simulink model "wlan_phy_tx_pmd"  (Simulink 7.8)
settings: Solver=ode45  StartTime=0.0  StopTime=17e3  RelTol=1e-3
PostLoadFcn:
  | wlan_phy_tx_init
InitFcn:
  | wlan_phy_tx_init
StartFcn:
  | wlan_phy_tx_init
undefined symbols (not defined in the file): gcbh, interleave_16QAM, interleave_64QAM_addr, interleave_bpsk, interleave_QPSK, MAX_NUM_BYTES, MAX_NUM_SC, Mod_Constellation_16QAM, Mod_Constellation_64QAM, Mod_Constellation_BPSK, Mod_Constellation_QPSK, Preamble_IQ, xlBlockLoadCallback, xlGetNormalizedPeriod
libraries: xbsIndex_r4 x1164, xbsEDKLib_r4 x1
(part 4 of 8)

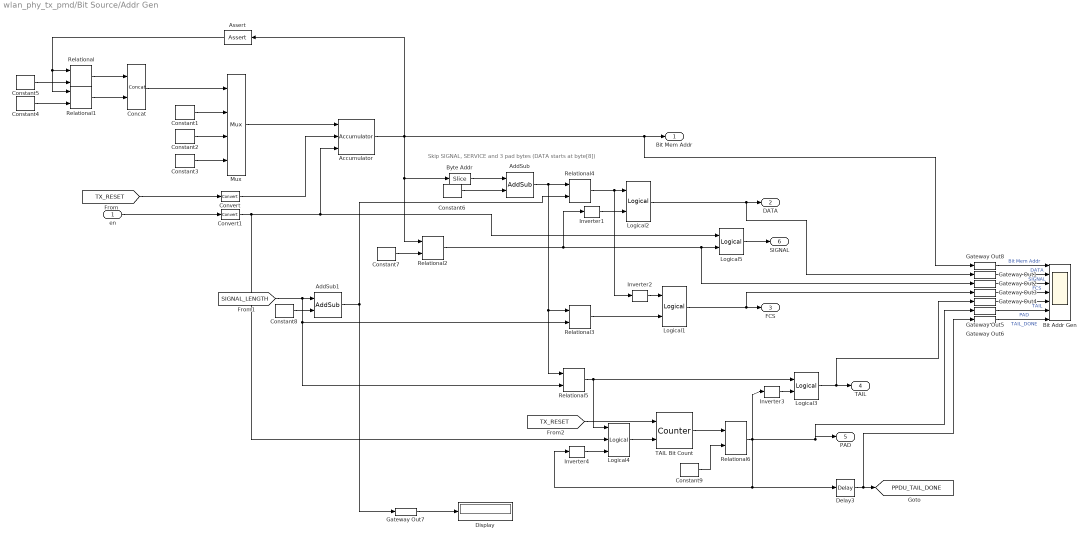
== system wlan_phy_tx_pmd/Bit Source/Addr Gen ==
  note: Skip SIGNAL, SERVICE and
      | 3 pad bytes
      | (DATA starts at byte[8])
  en : Inport
  Accumulator : xbsIndex_r4/Accumulator  operation=Add  n_bits=3 + ceil(log2(MAX_NUM_BYTES))  overflow=Wrap  scale=1  rst=on  infoeditControl=reset for floating point data type must be asserted for a minimum of 2 cycles  hasbypass=off  en=on  latency=0  dbl_ovrd=off  msb_inp=100  msb=100  lsb=-100  use_behavioral_HDL=on  implementation=Fabric  block_type=accum
  AddSub : xbsIndex_r4/AddSub  mode=Subtraction  use_carryin=off  use_carryout=off  en=off  latency=0  precision=User Defined  arith_type=Unsigned  n_bits=ceil(log2(MAX_NUM_BYTES))  bin_pt=0  quantization=Truncate  overflow=Saturate  dbl_ovrd=off  use_behavioral_HDL=off  hw_selection=Fabric  pipelined=off  block_type=addsub
  AddSub1 : xbsIndex_r4/AddSub  mode=Subtraction  use_carryin=off  use_carryout=off  en=off  latency=0  precision=User Defined  arith_type=Unsigned  n_bits=ceil(log2(MAX_NUM_BYTES))  bin_pt=0  quantization=Truncate  overflow=Saturate  dbl_ovrd=off  use_behavioral_HDL=off  hw_selection=Fabric  pipelined=off  block_type=addsub
  Assert : xbsIndex_r4/Assert  assert_type=off  type_source=Explicitly  gui_display_data_type=Fixed-point  arith_type="Signed  (2's comp)"  n_bits=16  bin_pt=14  preci_type=Single  exp_width=8  frac_width=24  assert_rate=on  rate_source=Explicitly  period=1  output_port=on  block_type=assert
  Bit Addr Gen : Scope  NumInputPorts=7
      settings: TimeRange=10000  YMin=0~0~0~0~0~0~0  YMax=1~1~1~1~25~1~1  SaveName=ScopeData8
  Byte Addr : xbsIndex_r4/Slice  nbits=ceil(log2(MAX_NUM_BYTES))  boolean_output=off  mode=Upper Bit Location + Width  bit1=0  base1=MSB of Input  bit0=0  base0=LSB of Input  dbl_ovrd=off  block_type=slice
  Concat : xbsIndex_r4/Concat  num_inputs=2  dbl_ovrd=off  block_type=concat
  Constant1 : xbsIndex_r4/Constant  const=1  gui_display_data_type=Fixed-point  arith_type=Unsigned  n_bits=2  bin_pt=0  preci_type=Single  exp_width=8  frac_width=24  explicit_period=off  period=1  equ=P=C  opselect=C  inp2=PCIN>>17  opr=+  inp1=P  carry=CIN  dbl_ovrd=off  block_type=constant
  Constant2 : xbsIndex_r4/Constant  const=9  gui_display_data_type=Fixed-point  arith_type=Unsigned  n_bits=4  bin_pt=0  preci_type=Single  exp_width=8  frac_width=24  explicit_period=off  period=1  equ=P=C  opselect=C  inp2=PCIN>>17  opr=+  inp1=P  carry=CIN  dbl_ovrd=off  block_type=constant
  Constant3 : xbsIndex_r4/Constant  const=17  gui_display_data_type=Fixed-point  arith_type=Unsigned  n_bits=5  bin_pt=0  preci_type=Single  exp_width=8  frac_width=24  explicit_period=off  period=1  equ=P=C  opselect=C  inp2=PCIN>>17  opr=+  inp1=P  carry=CIN  dbl_ovrd=off  block_type=constant
  Constant4 : xbsIndex_r4/Constant  const=23  gui_display_data_type=Fixed-point  arith_type=Unsigned  n_bits=5  bin_pt=0  preci_type=Single  exp_width=8  frac_width=24  explicit_period=off  period=1  equ=P=C  opselect=C  inp2=PCIN>>17  opr=+  inp1=P  carry=CIN  dbl_ovrd=off  block_type=constant
  Constant5 : xbsIndex_r4/Constant  const=47  gui_display_data_type=Fixed-point  arith_type=Unsigned  n_bits=6  bin_pt=0  preci_type=Single  exp_width=8  frac_width=24  explicit_period=off  period=1  equ=P=C  opselect=C  inp2=PCIN>>17  opr=+  inp1=P  carry=CIN  dbl_ovrd=off  block_type=constant
  Constant6 : xbsIndex_r4/Constant  const=8  gui_display_data_type=Fixed-point  arith_type=Unsigned  n_bits=4  bin_pt=0  preci_type=Single  exp_width=8  frac_width=24  explicit_period=off  period=1  equ=P=C  opselect=C  inp2=PCIN>>17  opr=+  inp1=P  carry=CIN  dbl_ovrd=off  block_type=constant
  Constant7 : xbsIndex_r4/Constant  const=24  gui_display_data_type=Fixed-point  arith_type=Unsigned  n_bits=5  bin_pt=0  preci_type=Single  exp_width=8  frac_width=24  explicit_period=off  period=1  equ=P=C  opselect=C  inp2=PCIN>>17  opr=+  inp1=P  carry=CIN  dbl_ovrd=off  block_type=constant
  Constant8 : xbsIndex_r4/Constant  const=4  gui_display_data_type=Fixed-point  arith_type=Unsigned  n_bits=3  bin_pt=0  preci_type=Single  exp_width=8  frac_width=24  explicit_period=off  period=1  equ=P=C  opselect=C  inp2=PCIN>>17  opr=+  inp1=P  carry=CIN  dbl_ovrd=off  block_type=constant
  Constant9 : xbsIndex_r4/Constant  const=5  gui_display_data_type=Fixed-point  arith_type=Unsigned  n_bits=3  bin_pt=0  preci_type=Single  exp_width=8  frac_width=24  explicit_period=off  period=1  equ=P=C  opselect=C  inp2=PCIN>>17  opr=+  inp1=P  carry=CIN  dbl_ovrd=off  block_type=constant
  Convert : xbsIndex_r4/Convert  gui_display_data_type=Boolean  arith_type=Boolean  n_bits=16  bin_pt=14  float_type=Single  exp_bits=8  fraction_bits=24  quantization=Truncate  overflow=Wrap  en=off  latency=0  dbl_ovrd=off  pipeline=off  block_type=convert
  Convert1 : xbsIndex_r4/Convert  gui_display_data_type=Boolean  arith_type=Boolean  n_bits=16  bin_pt=14  float_type=Single  exp_bits=8  fraction_bits=24  quantization=Truncate  overflow=Wrap  en=off  latency=0  dbl_ovrd=off  pipeline=off  block_type=convert
  Delay3 : xbsIndex_r4/Delay  rst=off  infoeditControl=Selection of Reset will increase slice count due to use of real FFs and instead of SRLs  en=off  latency=1  dbl_ovrd=off  reg_retiming=off  block_type=delay
  Display : Display
  Gateway Out{1..8} (8 alike) : xbsIndex_r4/Gateway Out  inherit_from_input=off  hdl_port=off  timing_constraint=None  locs_specified=off  LOCs={}  UseAsDAC=off  DACChannel='1'  block_type=gatewayout
  Inverter{1..4} (4 alike) : xbsIndex_r4/Inverter  en=off  latency=0  dbl_ovrd=off  block_type=inv
      settings: xl_area=[0 0 0 0 0 0 0]  block_version=VER_STRING_GOES_HERE
  Logical{1..3,5} (4 alike) : xbsIndex_r4/Logical  logical_function=AND  inputs=2  en=off  latency=0  precision=Full  arith_type=Unsigned  n_bits=16  bin_pt=0  align_bp=on  dbl_ovrd=off  block_type=logical
  Logical4 : xbsIndex_r4/Logical  logical_function=AND  inputs=3  en=off  latency=0  precision=Full  arith_type=Unsigned  n_bits=16  bin_pt=0  align_bp=on  dbl_ovrd=off  block_type=logical
  Mux : xbsIndex_r4/Mux  inputs=3  en=off  latency=0  precision=Full  arith_type=Unsigned  n_bits=16  bin_pt=14  quantization=Truncate  overflow=Wrap  dbl_ovrd=off  block_type=mux
  Relational : xbsIndex_r4/Relational  mode=a=b  en=off  latency=0  dbl_ovrd=off  block_type=relational
  Relational1 : xbsIndex_r4/Relational  mode=a=b  en=off  latency=0  dbl_ovrd=off  block_type=relational
  Relational2 : xbsIndex_r4/Relational  mode=a<b  en=off  latency=0  dbl_ovrd=off  block_type=relational
  Relational3 : xbsIndex_r4/Relational  mode=a<b  en=off  latency=0  dbl_ovrd=off  block_type=relational
  Relational4 : xbsIndex_r4/Relational  mode=a<b  en=off  latency=0  dbl_ovrd=off  block_type=relational
  Relational5 : xbsIndex_r4/Relational  mode=a>=b  en=off  latency=0  dbl_ovrd=off  block_type=relational
  Relational6 : xbsIndex_r4/Relational  mode=a>b  en=off  latency=0  dbl_ovrd=off  block_type=relational
  TAIL Bit Count : xbsIndex_r4/Counter  cnt_type=Count Limited  cnt_to=6  operation=Up  start_count=0  cnt_by_val=1  arith_type=Unsigned  n_bits=3  bin_pt=0  load_pin=off  rst=on  en=on  explicit_period=on  period=1  dbl_ovrd=off  use_behavioral_HDL=off  implementation=Fabric  block_type=counter
  Bit Mem Addr : Outport
  DATA : Outport  Port=2
  FCS : Outport  Port=3
  TAIL : Outport  Port=4
  PAD : Outport  Port=5
  SIGNAL : Outport  Port=6
  tag scope: PPDU_TAIL_DONE=global
  wires:
  Convert1/1 -> Logical4/2, Accumulator/3, Logical5/1
  Convert/1 -> Accumulator/2
  Assert/1 -> Relational1/1, Relational/1
  Relational1/1 -> Concat/2
  Relational/1 -> Concat/1
  Constant4/1 -> Relational1/2
  Constant5/1 -> Relational/2
  Accumulator/1 -> Assert/1, Byte Addr/1, Relational2/1, Bit Mem Addr/1, Gateway Out8/1
  [TX_RESET] -> Convert/1
  en/1 -> Convert1/1
  Mux/1 -> Accumulator/1
  Constant3/1 -> Mux/4
  Constant2/1 -> Mux/3
  Constant1/1 -> Mux/2
  Constant6/1 -> AddSub/2
  Byte Addr/1 -> AddSub/1
  AddSub/1 -> Relational4/1, Relational3/1, Relational5/1
  Concat/1 -> Mux/1
  Constant7/1 -> Relational2/2
  Relational2/1 -> Inverter1/1, Gateway Out2/1, Logical5/2
  AddSub1/1 -> Relational4/2, Gateway Out7/1
  Relational4/1 -> Logical2/1, Inverter2/1
  Inverter1/1 -> Logical2/2
  Logical2/1 -> DATA/1, Gateway Out1/1
  [SIGNAL_LENGTH] -> AddSub1/1, Relational3/2, Relational5/2
  Constant8/1 -> AddSub1/2
  Inverter2/1 -> Logical1/1
  Relational3/1 -> Logical1/2
  Logical1/1 -> FCS/1, Gateway Out3/1
  Relational5/1 -> Logical3/1, Logical4/1
  Inverter3/1 -> Logical3/2
  Logical3/1 -> TAIL/1, Gateway Out4/1
  Logical4/1 -> TAIL Bit Count/2
  [TX_RESET] -> TAIL Bit Count/1
  TAIL Bit Count/1 -> Relational6/1
  Relational6/1 -> Inverter3/1, PAD/1, Gateway Out5/1, Delay3/1, Inverter4/1
  Constant9/1 -> Relational6/2
  Delay3/1 -> [PPDU_TAIL_DONE], Gateway Out6/1
  Gateway Out8/1 -> Bit Addr Gen/1  "Bit Mem Addr"
  Gateway Out1/1 -> Bit Addr Gen/2  "DATA"
  Gateway Out2/1 -> Bit Addr Gen/3  "SIGNAL"
  Gateway Out3/1 -> Bit Addr Gen/4  "FCS"
  Gateway Out4/1 -> Bit Addr Gen/5  "TAIL"
  Gateway Out5/1 -> Bit Addr Gen/6  "PAD"
  Gateway Out6/1 -> Bit Addr Gen/7  "TAIL_DONE"
  Inverter4/1 -> Logical4/3
  Logical5/1 -> SIGNAL/1
  Gateway Out7/1 -> Display/1

== system wlan_phy_tx_pmd/Bit Source/BRAM IF 64b ==
  Bit Addr : Inport
  9MSB : xbsIndex_r4/Slice  nbits=9  boolean_output=off  mode=Upper Bit Location + Width  bit1=0  base1=MSB of Input  bit0=0  base0=LSB of Input  dbl_ovrd=off  block_type=slice
      settings: block_version=8.2.02
  AddSub : xbsIndex_r4/AddSub  mode=Addition  use_carryin=off  use_carryout=off  en=off  latency=0  precision=User Defined  arith_type=Unsigned  n_bits=9  bin_pt=0  quantization=Truncate  overflow=Wrap  dbl_ovrd=off  use_behavioral_HDL=off  hw_selection=Fabric  pipelined=off  block_type=addsub
  BRAM_Addr : xbsIndex_r4/Gateway Out  inherit_from_input=off  hdl_port=on  timing_constraint=None  locs_specified=off  LOCs={}  UseAsDAC=off  DACChannel='1'  block_type=gatewayout
      settings: infoedit="Gateway out block.  Converts Xilinx fixed point inputs into ouputs of type Simulink integer, double, or fixed point.<P><P>Hardware notes:  In hardware these blocks become top level output ports or are discarded, depending on how they are configured."  xl_area=[0, 0, 0, 0, 0, 0, 0]  block_version=VER_STRING_GOES_HERE
  BRAM_Din : xbsIndex_r4/Gateway In  gui_display_data_type=Fixed-point  arith_type=Unsigned  n_bits=64  bin_pt=0  preci_type=Single  exp_width=8  frac_width=24  quantization="Round  (unbiased: +/- Inf)"  overflow=Saturate  period=1  dbl_ovrd=off  timing_constraint=None  locs_specified=off  LOCs={}  UseAsADC=off  ADCChannel='1'  inherit_from_input=off  hdl_port=on  block_type=gatewayin
      settings: block_version=VER_STRING_GOES_HERE
  BRAM_Dout : xbsIndex_r4/Gateway Out  inherit_from_input=off  hdl_port=on  timing_constraint=None  locs_specified=off  LOCs={}  UseAsDAC=off  DACChannel='1'  block_type=gatewayout
      settings: infoedit="Gateway out block.  Converts Xilinx fixed point inputs into ouputs of type Simulink integer, double, or fixed point.<P><P>Hardware notes:  In hardware these blocks become top level output ports or are discarded, depending on how they are configured."  xl_area=[0, 0, 0, 0, 0, 0, 0]  block_version=VER_STRING_GOES_HERE
  BRAM_En : xbsIndex_r4/Gateway Out  inherit_from_input=off  hdl_port=on  timing_constraint=None  locs_specified=off  LOCs={}  UseAsDAC=off  DACChannel='1'  block_type=gatewayout
      settings: infoedit="Gateway out block.  Converts Xilinx fixed point inputs into ouputs of type Simulink integer, double, or fixed point.<P><P>Hardware notes:  In hardware these blocks become top level output ports or are discarded, depending on how they are configured."  block_version=8.2.02
  BRAM_Reset : xbsIndex_r4/Gateway Out  inherit_from_input=off  hdl_port=on  timing_constraint=None  locs_specified=off  LOCs={}  UseAsDAC=off  DACChannel='1'  block_type=gatewayout
      settings: infoedit="Gateway out block.  Converts Xilinx fixed point inputs into ouputs of type Simulink integer, double, or fixed point.<P><P>Hardware notes:  In hardware these blocks become top level output ports or are discarded, depending on how they are configured."  block_version=8.2.02
  BRAM_WEn : xbsIndex_r4/Gateway Out  inherit_from_input=off  hdl_port=on  timing_constraint=None  locs_specified=off  LOCs={}  UseAsDAC=off  DACChannel='1'  block_type=gatewayout
      settings: infoedit="Gateway out block.  Converts Xilinx fixed point inputs into ouputs of type Simulink integer, double, or fixed point.<P><P>Hardware notes:  In hardware these blocks become top level output ports or are discarded, depending on how they are configured."  xl_area=[0, 0, 0, 0, 0, 0, 0]  block_version=VER_STRING_GOES_HERE
  Concat : xbsIndex_r4/Concat  num_inputs=4  dbl_ovrd=off  block_type=concat
  Constant : Constant  Value=0
  Constant1 : xbsIndex_r4/Constant  const=1  gui_display_data_type=Fixed-point  arith_type=Unsigned  n_bits=1  bin_pt=0  preci_type=Single  exp_width=8  frac_width=24  explicit_period=on  period=1  equ=P=C  opselect=C  inp2=PCIN>>17  opr=+  inp1=P  carry=CIN  dbl_ovrd=off  block_type=constant
      settings: block_version=8.2.02
  Constant2 : xbsIndex_r4/Constant  const=0  gui_display_data_type=Fixed-point  arith_type=Unsigned  n_bits=1  bin_pt=0  preci_type=Single  exp_width=8  frac_width=24  explicit_period=on  period=1  equ=P=C  opselect=C  inp2=PCIN>>17  opr=+  inp1=P  carry=CIN  dbl_ovrd=off  block_type=constant
      settings: block_version=8.2.02
  Constant3 : xbsIndex_r4/Constant  const=0  gui_display_data_type=Fixed-point  arith_type=Unsigned  n_bits=3  bin_pt=0  preci_type=Single  exp_width=8  frac_width=24  explicit_period=off  period=1  equ=P=C  opselect=C  inp2=PCIN>>17  opr=+  inp1=P  carry=CIN  dbl_ovrd=off  block_type=constant
  Constant4 : xbsIndex_r4/Constant  const=0  gui_display_data_type=Fixed-point  arith_type=Unsigned  n_bits=16  bin_pt=0  preci_type=Single  exp_width=8  frac_width=24  explicit_period=off  period=1  equ=P=C  opselect=C  inp2=PCIN>>17  opr=+  inp1=P  carry=CIN  dbl_ovrd=off  block_type=constant
  Constant7 : xbsIndex_r4/Constant  const=0  gui_display_data_type=Fixed-point  arith_type=Unsigned  n_bits=64  bin_pt=0  preci_type=Single  exp_width=8  frac_width=24  explicit_period=on  period=1  equ=P=C  opselect=C  inp2=PCIN>>17  opr=+  inp1=P  carry=CIN  dbl_ovrd=off  block_type=constant
      settings: block_version=8.2.02
  Constant8 : xbsIndex_r4/Constant  const=0  gui_display_data_type=Fixed-point  arith_type=Unsigned  n_bits=8  bin_pt=0  preci_type=Single  exp_width=8  frac_width=24  explicit_period=on  period=1  equ=P=C  opselect=C  inp2=PCIN>>17  opr=+  inp1=P  carry=CIN  dbl_ovrd=off  block_type=constant
      settings: block_version=8.2.02
  Gateway Out1 : xbsIndex_r4/Gateway Out  inherit_from_input=off  hdl_port=off  timing_constraint=None  locs_specified=off  LOCs={}  UseAsDAC=off  DACChannel='1'  block_type=gatewayout
  Gateway Out8 : xbsIndex_r4/Gateway Out  inherit_from_input=off  hdl_port=off  timing_constraint=None  locs_specified=off  LOCs={}  UseAsDAC=off  DACChannel='1'  block_type=gatewayout
  Pkt Buf : Scope  NumInputPorts=7
      settings: TimeRange=30000  YMin=0~0~0~-0.1~0~-0.1~-0.1  YMax=300~300~1~1.1~4000~1.1~1.1  SaveName=ScopeData6
  Sim RAM : Subsystem
  Simulation Multiplexer : xbsIndex_r4/Simulation Multiplexer  sim_sel=1  hw_sel=2  block_type=simmux
      settings: infoedit="Distinguish input subsystems as \"simulation only\" and \"generation only\".  The input specified For Simulation will be used during Simulink simulation.  The input specified For Generation will be used during code generation.  This block will typically be used on the output of a HW Co-Simulation, Black Box, or ModelSim subsystem.<br><br>Hardware Notes: This block costs nothing."
  Terminator{,2..5} (5 alike) : Terminator
  64b Data : Outport
  wires:
  Concat/1 -> BRAM_Addr/1
  9MSB/1 -> AddSub/1
  [regTx_Pkt_Buf_Addr_Offset] -> AddSub/2
  [Tx_PKT_BUF_SEL] -> Concat/2
  Constant4/1 -> Concat/1
  Gateway Out1/1 -> Pkt Buf/2  "Data"
  Gateway Out8/1 -> Pkt Buf/1  "Addr"
  Constant3/1 -> Concat/4
  AddSub/1 -> Concat/3, Gateway Out8/1, Sim RAM/1(Addr)
  Constant8/1 -> BRAM_WEn/1
  Constant7/1 -> BRAM_Dout/1
  Constant/1 -> BRAM_Din/1
  Bit Addr/1 -> 9MSB/1
  Constant1/1 -> BRAM_En/1
  Constant2/1 -> BRAM_Reset/1
  BRAM_Addr/1 -> Terminator/1
  BRAM_Dout/1 -> Terminator2/1
  BRAM_En/1 -> Terminator3/1
  BRAM_Reset/1 -> Terminator4/1
  BRAM_WEn/1 -> Terminator5/1
  BRAM_Din/1 -> Simulation Multiplexer/2
  Simulation Multiplexer/1 -> 64b Data/1
  Sim RAM/1(64b) -> Gateway Out1/1, Simulation Multiplexer/1

== system wlan_phy_tx_pmd/Bit Source/Bit Per Sym Counter ==
  Start Sym : Inport
  Bit Src Sym Ctr : Scope  NumInputPorts=5
      settings: YMin=-5~-5~-5~-5~-5  YMax=5~5~5~5~5  SaveName=ScopeData10
  Constant2 : xbsIndex_r4/Constant  const=24  gui_display_data_type=Fixed-point  arith_type=Unsigned  n_bits=5  bin_pt=0  preci_type=Single  exp_width=8  frac_width=24  explicit_period=off  period=1  equ=P=C  opselect=C  inp2=PCIN>>17  opr=+  inp1=P  carry=CIN  dbl_ovrd=off  block_type=constant
  Gateway Out{1..4,14} (5 alike) : xbsIndex_r4/Gateway Out  inherit_from_input=off  hdl_port=off  timing_constraint=None  locs_specified=off  LOCs={}  UseAsDAC=off  DACChannel='1'  block_type=gatewayout
  Inverter : xbsIndex_r4/Inverter  en=off  latency=0  dbl_ovrd=off  block_type=inv
      settings: xl_area=[0 0 0 0 0 0 0]  block_version=VER_STRING_GOES_HERE
  Logical1 : xbsIndex_r4/Logical  logical_function=OR  inputs=2  en=off  latency=0  precision=Full  arith_type=Unsigned  n_bits=8  bin_pt=2  align_bp=on  dbl_ovrd=off  block_type=logical
      settings: xl_area=[1 0 0 1 0 0 0]  block_version=VER_STRING_GOES_HERE
  Logical2 : xbsIndex_r4/Logical  logical_function=OR  inputs=2  en=off  latency=0  precision=Full  arith_type=Unsigned  n_bits=8  bin_pt=2  align_bp=on  dbl_ovrd=off  block_type=logical
      settings: xl_area=[1 0 0 1 0 0 0]  block_version=VER_STRING_GOES_HERE
  Logical3 : xbsIndex_r4/Logical  logical_function=OR  inputs=2  en=off  latency=0  precision=Full  arith_type=Unsigned  n_bits=8  bin_pt=2  align_bp=on  dbl_ovrd=off  block_type=logical
      settings: xl_area=[1 0 0 1 0 0 0]  block_version=VER_STRING_GOES_HERE
  Mux : xbsIndex_r4/Mux  inputs=2  en=off  latency=0  precision=Full  arith_type=Unsigned  n_bits=16  bin_pt=14  quantization=Truncate  overflow=Wrap  dbl_ovrd=off  block_type=mux
  Osc : Subsystem
  Posedge1 : Subsystem
  Relational2 : xbsIndex_r4/Relational  mode=a<b  en=off  latency=0  dbl_ovrd=off  block_type=relational
  S-R Latch1 : Subsystem
  S-R Latch2 : Subsystem
  Sym Data Bit Count : xbsIndex_r4/Counter  cnt_type=Free Running  cnt_to=Inf  operation=Up  start_count=0  cnt_by_val=1  arith_type=Unsigned  n_bits=9  bin_pt=0  load_pin=off  rst=on  en=on  explicit_period=off  period=1  dbl_ovrd=off  use_behavioral_HDL=off  implementation=Fabric  block_type=counter
  Load Bit : Outport
  Last Bit in Sym : Outport  Port=2
  wires:
  [DATA_N_DBPS] -> Mux/3
  Constant2/1 -> Mux/2
  Mux/1 -> Relational2/2, Gateway Out4/1
  Sym Data Bit Count/1 -> Relational2/1, Gateway Out3/1
  Relational2/1 -> Inverter/1
  Inverter/1 -> Logical1/1, Logical2/2, S-R Latch2/1(S), Logical3/2, Last Bit in Sym/1, Gateway Out2/1
  [TX_RESET] -> Logical2/1, Logical1/2, S-R Latch2/2(R)
  Posedge1/1(Q) -> S-R Latch1/1(S)
  Start Sym/1 -> Posedge1/1(D)
  Logical1/1 -> Sym Data Bit Count/1
  Logical2/1 -> S-R Latch1/2(R)
  S-R Latch1/1(Q) -> Osc/2(En), Gateway Out14/1
  Osc/1(Q) -> Sym Data Bit Count/2, Load Bit/1, Gateway Out1/1
  S-R Latch2/1(Q) -> Mux/1
  Logical3/1 -> Osc/1(Rst)
  [TX_RESET] -> Logical3/1
  Gateway Out14/1 -> Bit Src Sym Ctr/1
  Gateway Out1/1 -> Bit Src Sym Ctr/2
  Gateway Out2/1 -> Bit Src Sym Ctr/3
  Gateway Out3/1 -> Bit Src Sym Ctr/4
  Gateway Out4/1 -> Bit Src Sym Ctr/5

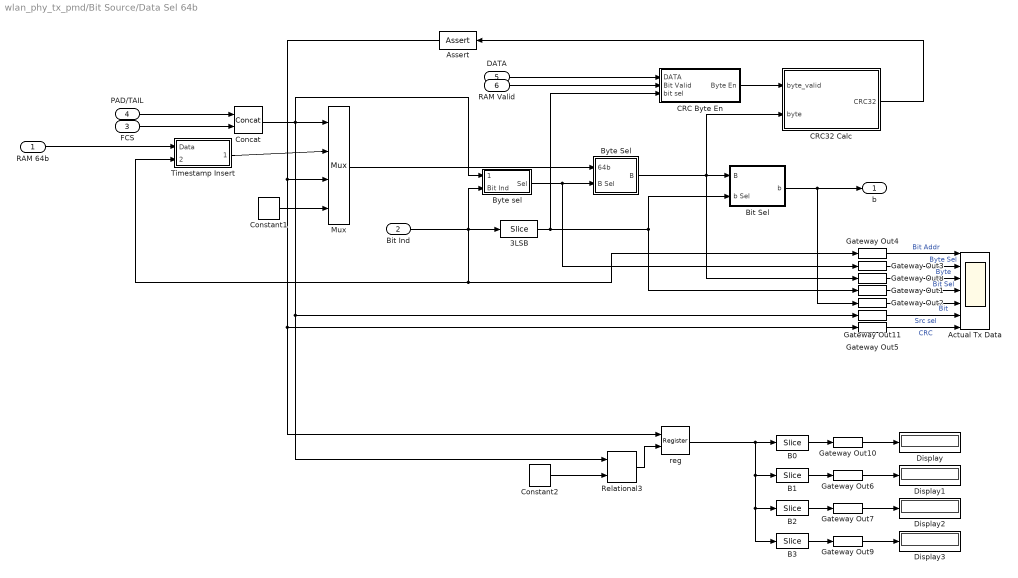
== system wlan_phy_tx_pmd/Bit Source/Data Sel 64b ==
  RAM 64b : Inport
  Bit Ind : Inport  Port=2
  FCS : Inport  Port=3
  PAD/TAIL : Inport  Port=4
  DATA : Inport  Port=5
  RAM Valid : Inport  Port=6
  3LSB : xbsIndex_r4/Slice  nbits=3  boolean_output=off  mode=Lower Bit Location + Width  bit1=0  base1=MSB of Input  bit0=0  base0=LSB of Input  dbl_ovrd=off  block_type=slice
      settings: block_version=8.2.02
  Actual Tx Data : Scope  NumInputPorts=7
      settings: TimeRange=18000  YMin=0~0~0~0~0~0~0  YMax=800~8~250~8~1~2~5000000000  SaveName=ScopeData14
  Assert : xbsIndex_r4/Assert  assert_type=off  type_source=Explicitly  gui_display_data_type=Fixed-point  arith_type="Signed  (2's comp)"  n_bits=16  bin_pt=14  preci_type=Single  exp_width=8  frac_width=24  assert_rate=on  rate_source=Explicitly  period=1  output_port=on  block_type=assert
  B0 : xbsIndex_r4/Slice  nbits=8  boolean_output=off  mode=Lower Bit Location + Width  bit1=0  base1=MSB of Input  bit0=0  base0=LSB of Input  dbl_ovrd=off  block_type=slice
  B1 : xbsIndex_r4/Slice  nbits=8  boolean_output=off  mode=Lower Bit Location + Width  bit1=0  base1=MSB of Input  bit0=8  base0=LSB of Input  dbl_ovrd=off  block_type=slice
  B2 : xbsIndex_r4/Slice  nbits=8  boolean_output=off  mode=Lower Bit Location + Width  bit1=0  base1=MSB of Input  bit0=16  base0=LSB of Input  dbl_ovrd=off  block_type=slice
  B3 : xbsIndex_r4/Slice  nbits=8  boolean_output=off  mode=Lower Bit Location + Width  bit1=0  base1=MSB of Input  bit0=24  base0=LSB of Input  dbl_ovrd=off  block_type=slice
  Bit Sel : Subsystem
  Byte Sel : Subsystem
  Byte sel : Subsystem
  CRC Byte En : Subsystem
  CRC32 Calc : Subsystem
  Concat : xbsIndex_r4/Concat  num_inputs=2  dbl_ovrd=off  block_type=concat
  Constant1 : xbsIndex_r4/Constant  const=0  gui_display_data_type=Fixed-point  arith_type=Unsigned  n_bits=32  bin_pt=0  preci_type=Single  exp_width=8  frac_width=24  explicit_period=off  period=1  equ=P=C  opselect=C  inp2=PCIN>>17  opr=+  inp1=P  carry=CIN  dbl_ovrd=off  block_type=constant
      settings: block_version=VER_STRING_GOES_HERE
  Constant2 : xbsIndex_r4/Constant  const=1  gui_display_data_type=Fixed-point  arith_type=Unsigned  n_bits=32  bin_pt=0  preci_type=Single  exp_width=8  frac_width=24  explicit_period=off  period=1  equ=P=C  opselect=C  inp2=PCIN>>17  opr=+  inp1=P  carry=CIN  dbl_ovrd=off  block_type=constant
      settings: block_version=VER_STRING_GOES_HERE
  Display{,1..3} (4 alike) : Display
  Gateway Out{1..11} (11 alike) : xbsIndex_r4/Gateway Out  inherit_from_input=off  hdl_port=off  timing_constraint=None  locs_specified=off  LOCs={}  UseAsDAC=off  DACChannel='1'  block_type=gatewayout
  Mux : xbsIndex_r4/Mux  inputs=3  en=off  latency=0  precision=Full  arith_type=Unsigned  n_bits=16  bin_pt=14  quantization=Truncate  overflow=Wrap  dbl_ovrd=off  block_type=mux
  Relational3 : xbsIndex_r4/Relational  mode=a=b  en=off  latency=0  dbl_ovrd=off  block_type=relational
  Timestamp Insert : Subsystem
  reg : xbsIndex_r4/Register  init=0  rst=off  en=on  dbl_ovrd=off  block_type=register
      settings: xl_area=[0, 0, 0, 0, 0, 0, 0]  block_version=VER_STRING_GOES_HERE
  b : Outport
  wires:
  CRC Byte En/1(Byte En) -> CRC32 Calc/1(byte_valid)
  RAM Valid/1 -> CRC Byte En/2(Bit Valid)
  DATA/1 -> CRC Byte En/1(DATA)
  Relational3/1 -> reg/2
  Constant2/1 -> Relational3/2
  reg/1 -> B3/1, B2/1, B1/1, B0/1
  Gateway Out11/1 -> Actual Tx Data/6  "Src sel"
  B1/1 -> Gateway Out6/1
  B2/1 -> Gateway Out7/1
  B3/1 -> Gateway Out9/1
  Gateway Out9/1 -> Display3/1
  Gateway Out7/1 -> Display2/1
  Gateway Out6/1 -> Display1/1
  Gateway Out10/1 -> Display/1
  B0/1 -> Gateway Out10/1
  Gateway Out5/1 -> Actual Tx Data/7  "CRC"
  Gateway Out4/1 -> Actual Tx Data/1  "Bit Addr"
  Gateway Out3/1 -> Actual Tx Data/2  "Byte Sel"
  Gateway Out2/1 -> Actual Tx Data/5  "Bit"
  Gateway Out1/1 -> Actual Tx Data/4  "Bit Sel"
  Gateway Out8/1 -> Actual Tx Data/3  "Byte"
  Assert/1 -> reg/1, Gateway Out5/1, Mux/3
  PAD/TAIL/1 -> Concat/1
  Constant1/1 -> Mux/4
  CRC32 Calc/1(CRC32) -> Assert/1
  FCS/1 -> Concat/2
  Concat/1 -> Byte sel/1(Src Sel), Relational3/1, Gateway Out11/1, Mux/1
  Bit Sel/1(b) -> Gateway Out2/1, b/1
  Mux/1 -> Byte Sel/1(64b)
  Byte sel/1(Sel) -> Gateway Out3/1, Byte Sel/2(B Sel)
  Bit Ind/1 -> Byte sel/2(Bit Ind), 3LSB/1, Gateway Out4/1, Timestamp Insert/2(Bit Ind)
  3LSB/1 -> CRC Byte En/3(bit sel), Bit Sel/2(b Sel), Gateway Out1/1
  Byte Sel/1(B) -> Gateway Out8/1, CRC32 Calc/2(byte), Bit Sel/1(B)
  Timestamp Insert/1(Tx Data) -> Mux/2
  RAM 64b/1 -> Timestamp Insert/1(Data)

== system wlan_phy_tx_pmd/Bit Source/Posedge ==
  D : Inport
  Delay : xbsIndex_r4/Delay  rst=off  infoeditControl=Selection of Reset will increase slice count due to use of real FFs and instead of SRLs  en=off  latency=1  dbl_ovrd=off  reg_retiming=off  block_type=delay
      settings: infoedit=Hardware notes: A delay line is a chain, each link of which is an SRL16 followed by a flip-flop. If register retiming is enabled, the delay line is a chain of flip-flops.  xl_area=[1 1 0 0 0 0 0]  block_version=VER_STRING_GOES_HERE
  Inverter : xbsIndex_r4/Inverter  en=off  latency=0  dbl_ovrd=off  block_type=inv
      settings: xl_area=[0 0 0 0 0 0 0]  block_version=VER_STRING_GOES_HERE
  Logical1 : xbsIndex_r4/Logical  logical_function=AND  inputs=2  en=off  latency=0  precision=Full  arith_type=Unsigned  n_bits=8  bin_pt=2  align_bp=on  dbl_ovrd=off  block_type=logical
      settings: xl_area=[1 0 0 1 0 0 0]  block_version=VER_STRING_GOES_HERE
  Q : Outport
  wires:
  D/1 -> Logical1/2, Delay/1
  Logical1/1 -> Q/1
  Inverter/1 -> Logical1/1
  Delay/1 -> Inverter/1

== system wlan_phy_tx_pmd/Bit Source/S-R Latch ==
  S : Inport
  R : Inport  Port=2
  Constant1 : xbsIndex_r4/Constant  const=1  gui_display_data_type=Fixed-point  arith_type=Boolean  n_bits=1  bin_pt=0  preci_type=Single  exp_width=8  frac_width=24  explicit_period=off  period=1  equ=P=C  opselect=C  inp2=PCIN>>17  opr=+  inp1=P  carry=CIN  dbl_ovrd=off  block_type=constant
      settings: block_version=VER_STRING_GOES_HERE
  Convert1 : xbsIndex_r4/Convert  gui_display_data_type=Boolean  arith_type=Boolean  n_bits=1  bin_pt=0  float_type=Single  exp_bits=8  fraction_bits=24  quantization=Truncate  overflow=Wrap  en=off  latency=0  dbl_ovrd=off  pipeline=off  block_type=convert
  Convert2 : xbsIndex_r4/Convert  gui_display_data_type=Boolean  arith_type=Boolean  n_bits=1  bin_pt=0  float_type=Single  exp_bits=8  fraction_bits=24  quantization=Truncate  overflow=Wrap  en=off  latency=0  dbl_ovrd=off  pipeline=off  block_type=convert
  Register2 : xbsIndex_r4/Register  init=0  rst=on  en=on  dbl_ovrd=off  block_type=register
      settings: xl_area=[1 1 0 0 0 0 0]  block_version=VER_STRING_GOES_HERE
  Q : Outport
  wires:
  Convert2/1 -> Register2/3
  Convert1/1 -> Register2/2
  Constant1/1 -> Register2/1
  R/1 -> Convert1/1
  Register2/1 -> Q/1
  S/1 -> Convert2/1

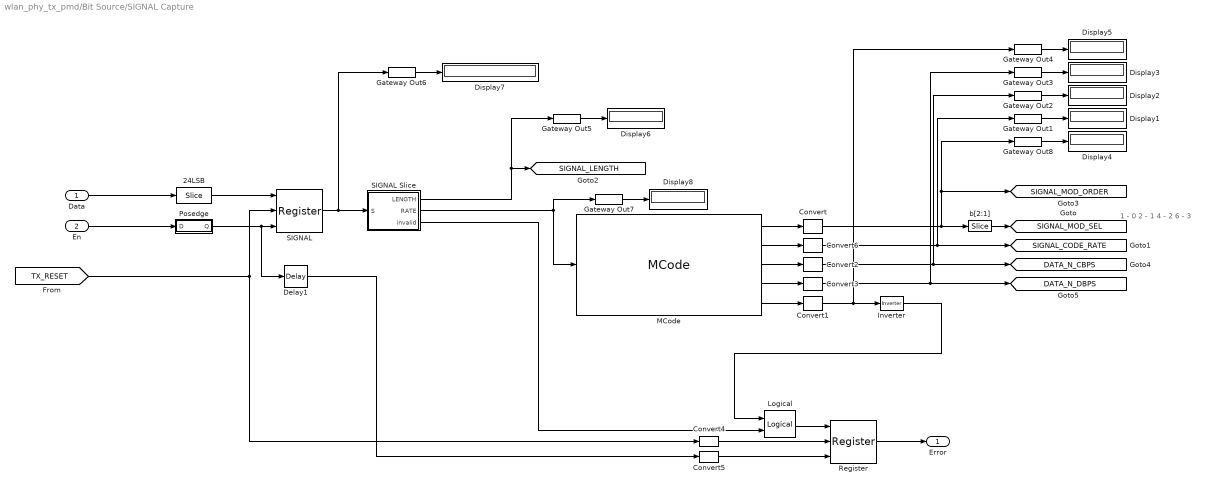
== system wlan_phy_tx_pmd/Bit Source/SIGNAL Capture ==
  note: 1 - 0
      | 2 - 1
      | 4 - 2
      | 6 - 3
  Data : Inport
  En : Inport  Port=2
  24LSB : xbsIndex_r4/Slice  nbits=24  boolean_output=off  mode=Lower Bit Location + Width  bit1=0  base1=MSB of Input  bit0=0  base0=LSB of Input  dbl_ovrd=off  block_type=slice
      settings: block_version=8.2.02
  Convert : xbsIndex_r4/Convert  gui_display_data_type=Fixed-point  arith_type=Unsigned  n_bits=4  bin_pt=0  float_type=Single  exp_bits=8  fraction_bits=24  quantization=Truncate  overflow=Wrap  en=off  latency=0  dbl_ovrd=off  pipeline=off  block_type=convert
  Convert1 : xbsIndex_r4/Convert  gui_display_data_type=Boolean  arith_type=Boolean  n_bits=1  bin_pt=0  float_type=Single  exp_bits=8  fraction_bits=24  quantization=Truncate  overflow=Wrap  en=off  latency=0  dbl_ovrd=off  pipeline=off  block_type=convert
  Convert2 : xbsIndex_r4/Convert  gui_display_data_type=Fixed-point  arith_type=Unsigned  n_bits=9  bin_pt=0  float_type=Single  exp_bits=8  fraction_bits=24  quantization=Truncate  overflow=Wrap  en=off  latency=0  dbl_ovrd=off  pipeline=off  block_type=convert
  Convert3 : xbsIndex_r4/Convert  gui_display_data_type=Fixed-point  arith_type=Unsigned  n_bits=9  bin_pt=0  float_type=Single  exp_bits=8  fraction_bits=24  quantization=Truncate  overflow=Wrap  en=off  latency=0  dbl_ovrd=off  pipeline=off  block_type=convert
  Convert4 : xbsIndex_r4/Convert  gui_display_data_type=Boolean  arith_type=Boolean  n_bits=16  bin_pt=14  float_type=Single  exp_bits=8  fraction_bits=24  quantization=Truncate  overflow=Wrap  en=off  latency=0  dbl_ovrd=off  pipeline=off  block_type=convert
  Convert5 : xbsIndex_r4/Convert  gui_display_data_type=Boolean  arith_type=Boolean  n_bits=16  bin_pt=14  float_type=Single  exp_bits=8  fraction_bits=24  quantization=Truncate  overflow=Wrap  en=off  latency=0  dbl_ovrd=off  pipeline=off  block_type=convert
  Convert6 : xbsIndex_r4/Convert  gui_display_data_type=Fixed-point  arith_type=Unsigned  n_bits=2  bin_pt=0  float_type=Single  exp_bits=8  fraction_bits=24  quantization=Truncate  overflow=Wrap  en=off  latency=0  dbl_ovrd=off  pipeline=off  block_type=convert
  Delay1 : xbsIndex_r4/Delay  rst=off  infoeditControl=Selection of Reset will increase slice count due to use of real FFs and instead of SRLs  en=off  latency=1  dbl_ovrd=off  reg_retiming=off  block_type=delay
  Display{1..8} (8 alike) : Display
  Gateway Out{1..8} (8 alike) : xbsIndex_r4/Gateway Out  inherit_from_input=off  hdl_port=off  timing_constraint=None  locs_specified=off  LOCs={}  UseAsDAC=off  DACChannel='1'  block_type=gatewayout
  Inverter : xbsIndex_r4/Inverter  en=off  latency=0  dbl_ovrd=off  block_type=inv
  Logical : xbsIndex_r4/Logical  logical_function=OR  inputs=2  en=off  latency=0  precision=Full  arith_type=Unsigned  n_bits=16  bin_pt=0  align_bp=on  dbl_ovrd=off  block_type=logical
  MCode : xbsIndex_r4/MCode  mfname=signal_rate_decode_tx  explicit_period=off  period=1  inputsTable={'boundInpExpr'=>[''],'inputs'=>['signal_rate']}  outputsTable={'outputs'=>['mod_order','code_rate','N_CBPS','N_DBPS','valid'],'suppressOut'=>['off','off','off','off','off']}  dbl_ovrd=off  enable_stdout=off  enable_debug=off  suppress_output=on  defparams={}  hide_port_list={}  block_type=mcode
  Posedge : Subsystem
  Register : xbsIndex_r4/Register  init=0  rst=on  en=on  dbl_ovrd=off  block_type=register
  SIGNAL : xbsIndex_r4/Register  init=TX_SIGNAL_INIT_VALUE  rst=on  en=on  dbl_ovrd=off  block_type=register
  SIGNAL Slice : Subsystem
  b[2:1] : xbsIndex_r4/Slice  nbits=2  boolean_output=off  mode=Lower Bit Location + Width  bit1=0  base1=MSB of Input  bit0=1  base0=LSB of Input  dbl_ovrd=off  block_type=slice
      settings: block_version=8.2.02
  Error : Outport
  tag scope: DATA_N_CBPS=global, DATA_N_DBPS=global, SIGNAL_CODE_RATE=global, SIGNAL_LENGTH=global, SIGNAL_MOD_ORDER=global, SIGNAL_MOD_SEL=global
  wires:
  En/1 -> Posedge/1(D)
  24LSB/1 -> SIGNAL/1
  Data/1 -> 24LSB/1
  [TX_RESET] -> SIGNAL/2, Convert4/1
  SIGNAL/1 -> SIGNAL Slice/1(S), Gateway Out6/1
  SIGNAL Slice/2(RATE) -> MCode/1, Gateway Out7/1
  SIGNAL Slice/1(LENGTH) -> [SIGNAL_LENGTH], Gateway Out5/1
  MCode/1 -> Convert/1
  MCode/2 -> Convert6/1
  Convert/1 -> b[2:1]/1, [SIGNAL_MOD_ORDER], Gateway Out8/1
  Inverter/1 -> Logical/1
  MCode/5 -> Convert1/1
  b[2:1]/1 -> [SIGNAL_MOD_SEL]
  MCode/3 -> Convert2/1
  Convert2/1 -> [DATA_N_CBPS], Gateway Out2/1
  MCode/4 -> Convert3/1
  Convert3/1 -> [DATA_N_DBPS], Gateway Out3/1
  Register/1 -> Error/1
  Logical/1 -> Register/1
  Convert4/1 -> Register/2
  Convert5/1 -> Register/3
  Posedge/1(Q) -> SIGNAL/3, Delay1/1
  SIGNAL Slice/3(invalid) -> Logical/2
  Delay1/1 -> Convert5/1
  Gateway Out8/1 -> Display4/1
  Convert1/1 -> Inverter/1, Gateway Out4/1
  Convert6/1 -> [SIGNAL_CODE_RATE], Gateway Out1/1
  Gateway Out1/1 -> Display1/1
  Gateway Out2/1 -> Display2/1
  Gateway Out3/1 -> Display3/1
  Gateway Out4/1 -> Display5/1
  Gateway Out5/1 -> Display6/1
  Gateway Out6/1 -> Display7/1
  Gateway Out7/1 -> Display8/1

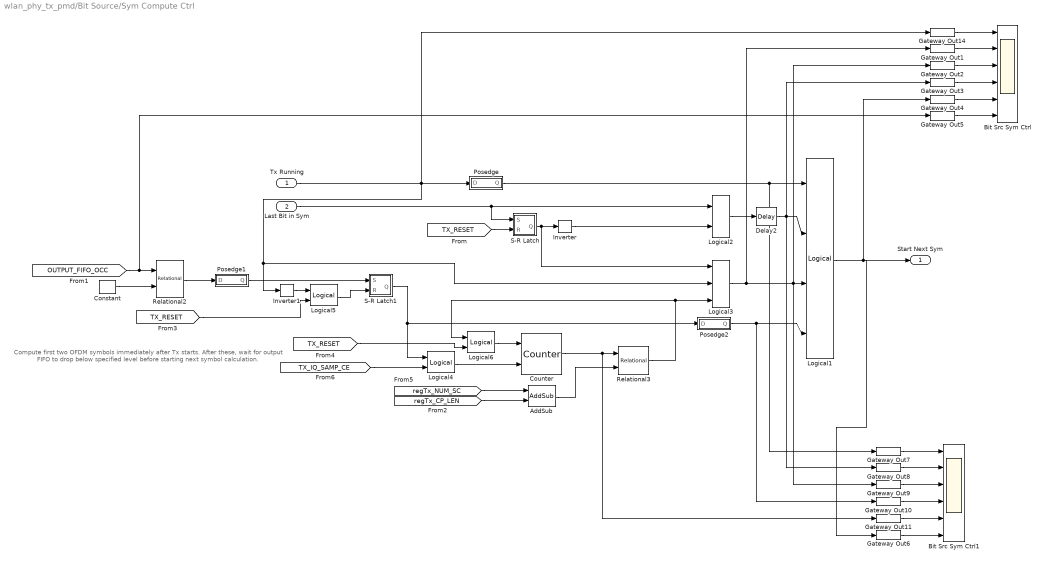
== system wlan_phy_tx_pmd/Bit Source/Sym Compute Ctrl ==
  note: Compute first two OFDM symbols immediately
      | after Tx starts. After these, wait for output FIFO
      | to drop below specified level before starting
      | next symbol calculation.
  Tx Running : Inport
  Last Bit in Sym : Inport  Port=2
  AddSub : xbsIndex_r4/AddSub  mode=Addition  use_carryin=off  use_carryout=off  en=off  latency=0  precision=Full  arith_type=Unsigned  n_bits=16  bin_pt=14  quantization=Truncate  overflow=Wrap  dbl_ovrd=off  use_behavioral_HDL=off  hw_selection=Fabric  pipelined=off  block_type=addsub
  Bit Src Sym Ctrl : Scope  NumInputPorts=6
      settings: YMin=0.95~0~0~-1~0~0  YMax=1.05~1~1~1~1~175  SaveName=ScopeData9
  Bit Src Sym Ctrl1 : Scope  NumInputPorts=6
      settings: YMin=0.95~0~0~-1~0~0  YMax=1.05~1~1~1~1~175  SaveName=ScopeData27
  Constant : xbsIndex_r4/Constant  const=120  gui_display_data_type=Fixed-point  arith_type=Unsigned  n_bits=8  bin_pt=0  preci_type=Single  exp_width=8  frac_width=24  explicit_period=off  period=1  equ=P=C  opselect=C  inp2=PCIN>>17  opr=+  inp1=P  carry=CIN  dbl_ovrd=off  block_type=constant
  Counter : xbsIndex_r4/Counter  cnt_type=Free Running  cnt_to=47  operation=Up  start_count=0  cnt_by_val=1  arith_type=Unsigned  n_bits=ceil(1+log2(MAX_NUM_SC))  bin_pt=0  load_pin=off  rst=on  en=on  explicit_period=off  period=4  dbl_ovrd=off  use_behavioral_HDL=off  implementation=Fabric  block_type=counter
  Delay2 : xbsIndex_r4/Delay  rst=off  infoeditControl=Selection of Reset will increase slice count due to use of real FFs and instead of SRLs  en=off  latency=80  dbl_ovrd=off  reg_retiming=off  block_type=delay
  Gateway Out{1..11,14} (12 alike) : xbsIndex_r4/Gateway Out  inherit_from_input=off  hdl_port=off  timing_constraint=None  locs_specified=off  LOCs={}  UseAsDAC=off  DACChannel='1'  block_type=gatewayout
  Inverter : xbsIndex_r4/Inverter  en=off  latency=0  dbl_ovrd=off  block_type=inv
      settings: xl_area=[0 0 0 0 0 0 0]  block_version=VER_STRING_GOES_HERE
  Inverter1 : xbsIndex_r4/Inverter  en=off  latency=0  dbl_ovrd=off  block_type=inv
      settings: xl_area=[0 0 0 0 0 0 0]  block_version=VER_STRING_GOES_HERE
  Logical1 : xbsIndex_r4/Logical  logical_function=OR  inputs=4  en=off  latency=0  precision=Full  arith_type=Unsigned  n_bits=8  bin_pt=2  align_bp=on  dbl_ovrd=off  block_type=logical
      settings: xl_area=[1 0 0 1 0 0 0]  block_version=VER_STRING_GOES_HERE
  Logical2 : xbsIndex_r4/Logical  logical_function=AND  inputs=2  en=off  latency=0  precision=Full  arith_type=Unsigned  n_bits=8  bin_pt=2  align_bp=on  dbl_ovrd=off  block_type=logical
      settings: xl_area=[1 0 0 1 0 0 0]  block_version=VER_STRING_GOES_HERE
  Logical3 : xbsIndex_r4/Logical  logical_function=AND  inputs=3  en=off  latency=0  precision=Full  arith_type=Unsigned  n_bits=8  bin_pt=2  align_bp=on  dbl_ovrd=off  block_type=logical
      settings: xl_area=[1 0 0 1 0 0 0]  block_version=VER_STRING_GOES_HERE
  Logical4 : xbsIndex_r4/Logical  logical_function=AND  inputs=2  en=off  latency=0  precision=Full  arith_type=Unsigned  n_bits=8  bin_pt=2  align_bp=on  dbl_ovrd=off  block_type=logical
      settings: xl_area=[1 0 0 1 0 0 0]  block_version=VER_STRING_GOES_HERE
  Logical5 : xbsIndex_r4/Logical  logical_function=OR  inputs=2  en=off  latency=0  precision=Full  arith_type=Unsigned  n_bits=8  bin_pt=2  align_bp=on  dbl_ovrd=off  block_type=logical
      settings: xl_area=[1 0 0 1 0 0 0]  block_version=VER_STRING_GOES_HERE
  Logical6 : xbsIndex_r4/Logical  logical_function=OR  inputs=2  en=off  latency=0  precision=Full  arith_type=Unsigned  n_bits=8  bin_pt=2  align_bp=on  dbl_ovrd=off  block_type=logical
      settings: xl_area=[1 0 0 1 0 0 0]  block_version=VER_STRING_GOES_HERE
  Posedge : Subsystem
  Posedge1 : Subsystem
  Posedge2 : Subsystem
  Relational2 : xbsIndex_r4/Relational  mode=a<b  en=off  latency=0  dbl_ovrd=off  block_type=relational
  Relational3 : xbsIndex_r4/Relational  mode=a=b  en=off  latency=0  dbl_ovrd=off  block_type=relational
  S-R Latch : Subsystem
  S-R Latch1 : Subsystem
  Start Next Sym : Outport
  wires:
  Tx Running/1 -> Posedge/1(D), Gateway Out14/1, Logical3/2, Inverter1/1
  Posedge/1(Q) -> Logical1/1, Gateway Out7/1
  [OUTPUT_FIFO_OCC] -> Relational2/1, Gateway Out5/1
  Constant/1 -> Relational2/2
  Relational2/1 -> Posedge1/1(D)
  Last Bit in Sym/1 -> S-R Latch/1(S), Logical2/1
  S-R Latch/1(Q) -> Inverter/1, Logical3/1
  [TX_RESET] -> S-R Latch/2(R)
  Logical2/1 -> Delay2/1
  Logical3/1 -> Gateway Out1/1, Logical1/3, Gateway Out2/1, Gateway Out9/1
  Delay2/1 -> Logical1/2, Gateway Out3/1, Gateway Out8/1
  Gateway Out14/1 -> Bit Src Sym Ctrl/1
  Gateway Out1/1 -> Bit Src Sym Ctrl/2
  Gateway Out2/1 -> Bit Src Sym Ctrl/3
  Gateway Out3/1 -> Bit Src Sym Ctrl/4
  Gateway Out4/1 -> Bit Src Sym Ctrl/5
  Inverter/1 -> Logical2/2
  [regTx_NUM_SC] -> AddSub/1
  [regTx_CP_LEN] -> AddSub/2
  Posedge1/1(Q) -> S-R Latch1/1(S)
  Counter/1 -> Relational3/1, Gateway Out11/1
  AddSub/1 -> Relational3/2
  Relational3/1 -> Logical3/3, Logical6/1
  [TX_IQ_SAMP_CE] -> Logical4/2
  Logical4/1 -> Counter/2
  S-R Latch1/1(Q) -> Posedge2/1(D), Logical4/1
  Gateway Out5/1 -> Bit Src Sym Ctrl/6
  Posedge2/1(Q) -> Logical1/4, Gateway Out10/1
  Logical1/1 -> Gateway Out4/1, Start Next Sym/1, Gateway Out6/1
  Gateway Out6/1 -> Bit Src Sym Ctrl1/6
  Gateway Out7/1 -> Bit Src Sym Ctrl1/1
  Gateway Out8/1 -> Bit Src Sym Ctrl1/2
  Gateway Out9/1 -> Bit Src Sym Ctrl1/3
  Logical5/1 -> S-R Latch1/2(R)
  Inverter1/1 -> Logical5/1
  [TX_RESET] -> Logical5/2
  Gateway Out10/1 -> Bit Src Sym Ctrl1/4
  Gateway Out11/1 -> Bit Src Sym Ctrl1/5
  Logical6/1 -> Counter/1
  [TX_RESET] -> Logical6/2

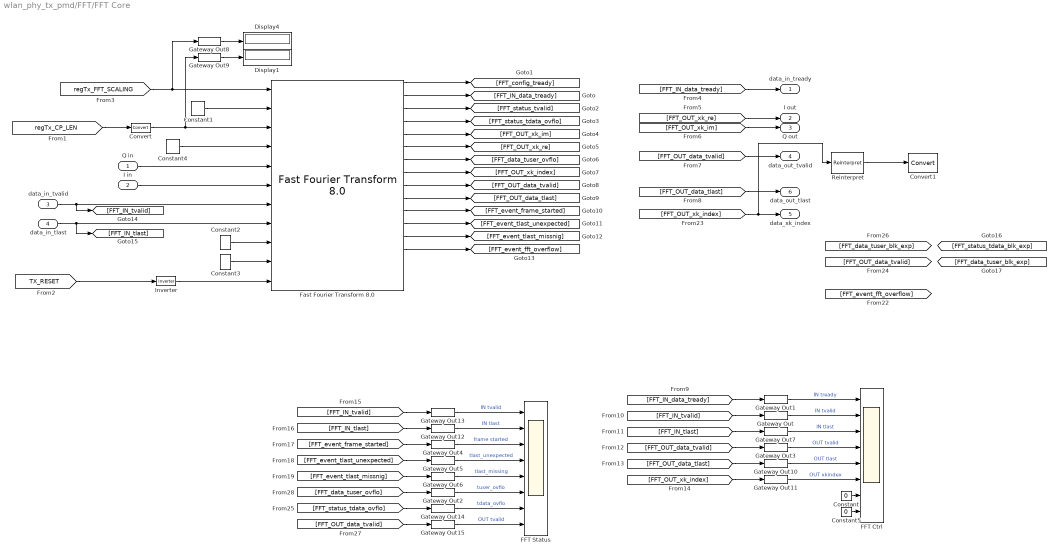
== system wlan_phy_tx_pmd/FFT/FFT Core ==
  Q in : Inport
  I in : Inport  Port=2
  data_in_tvalid : Inport  Port=3
  data_in_tlast : Inport  Port=4
  Constant : Constant  Value=0
  Constant1 : xbsIndex_r4/Constant  const=0  gui_display_data_type=Fixed-point  arith_type=Unsigned  n_bits=1  bin_pt=0  preci_type=Single  exp_width=8  frac_width=24  explicit_period=on  period=1  equ=P=C  opselect=C  inp2=PCIN>>17  opr=+  inp1=P  carry=CIN  dbl_ovrd=off  block_type=constant
  Constant2 : xbsIndex_r4/Constant  const=1  gui_display_data_type=Boolean  arith_type=Boolean  n_bits=1  bin_pt=0  preci_type=Single  exp_width=8  frac_width=24  explicit_period=on  period=1  equ=P=C  opselect=C  inp2=PCIN>>17  opr=+  inp1=P  carry=CIN  dbl_ovrd=off  block_type=constant
  Constant3 : xbsIndex_r4/Constant  const=1  gui_display_data_type=Boolean  arith_type=Boolean  n_bits=1  bin_pt=0  preci_type=Single  exp_width=8  frac_width=24  explicit_period=on  period=1  equ=P=C  opselect=C  inp2=PCIN>>17  opr=+  inp1=P  carry=CIN  dbl_ovrd=off  block_type=constant
  Constant4 : xbsIndex_r4/Constant  const=1  gui_display_data_type=Boolean  arith_type=Boolean  n_bits=1  bin_pt=0  preci_type=Single  exp_width=8  frac_width=24  explicit_period=on  period=1  equ=P=C  opselect=C  inp2=PCIN>>17  opr=+  inp1=P  carry=CIN  dbl_ovrd=off  block_type=constant
  Constant5 : Constant  Value=0
  Convert : xbsIndex_r4/Convert  gui_display_data_type=Fixed-point  arith_type=Unsigned  n_bits=6  bin_pt=0  float_type=Single  exp_bits=8  fraction_bits=24  quantization=Truncate  overflow=Wrap  en=off  latency=0  dbl_ovrd=off  pipeline=off  block_type=convert
  Convert1 : xbsIndex_r4/Convert  gui_display_data_type=Fixed-point  arith_type="Signed  (2's comp)"  n_bits=16  bin_pt=15  float_type=Single  exp_bits=8  fraction_bits=24  quantization=Truncate  overflow=Wrap  en=off  latency=0  dbl_ovrd=off  pipeline=off  block_type=convert
  Display1 : Display
  Display4 : Display
  FFT Ctrl : Scope  NumInputPorts=8
      settings: TimeRange=10000  YMin=0~0~-1~-1~0~-1~-1~0  YMax=1~1~1~1~1~1~1~1  SaveName=ScopeData12
  FFT Status : Scope  NumInputPorts=8
      settings: TimeRange=10000  YMin=0~0~0~-1~-1~0~0~0  YMax=1~1~1~1~1~6~6~1  SaveName=ScopeData13
  "Fast Fourier Transform 8.0 " : xbsIndex_r4/Fast Fourier Transform 8.0   transform_length=64  target_clock_frequency=160  target_data_throughput=50  implementation_options=radix_4_burst_io  run_time_configurable_transform_length=off  phase_factor_width=16  scaling_options=scaled  rounding_modes=truncation  aclken=off  aresetn=on  cyclic_prefix_insertion=on  output_ordering=natural_order  throttle_scheme=nonrealtime  xk_index=on  ovflo=on  trim_axipin_name=on  memory_options_data=block_ram  memory_options_phase_factors=block_ram  number_of_stages_using_block_ram_for_data_and_phase_factors=0  memory_options_reorder=block_ram  memory_options_hybrid=off  complex_mult_type=use_mults_performance  butterfly_type=use_luts  channels=1  input_ordering=natural_order  input_width=16  ip_name=Fast Fourier Transform  ip_version=8.0  dsptool_ready=true  ipcore_usecache=true  ipcore_useipmodelcache=true  wrapper_available=true  port_translation_map={ 'aclken' => 'en', 'aresetn' => 'rst'}  block_type=xfft_v8_0
  Gateway Out{,1..15} (16 alike) : xbsIndex_r4/Gateway Out  inherit_from_input=off  hdl_port=off  timing_constraint=None  locs_specified=off  LOCs={}  UseAsDAC=off  DACChannel='1'  block_type=gatewayout
  Inverter : xbsIndex_r4/Inverter  en=off  latency=0  dbl_ovrd=off  block_type=inv
  Reinterpret : xbsIndex_r4/Reinterpret  force_arith_type=off  arith_type=Unsigned  force_bin_pt=on  bin_pt=6  block_type=reinterpret
  data_in_tready : Outport
  I out : Outport  Port=2
  Q out : Outport  Port=3
  data_out_tvalid : Outport  Port=4
  data_xk_index : Outport  Port=5
  data_out_tlast : Outport  Port=6
  wires:
  Gateway Out8/1 -> Display4/1
  [regTx_CP_LEN] -> Convert/1
  [regTx_FFT_SCALING] -> Gateway Out8/1, "Fast Fourier Transform 8.0 "/1
  [TX_RESET] -> Inverter/1
  Gateway Out9/1 -> Display1/1
  data_in_tvalid/1 -> [FFT_IN_tvalid], "Fast Fourier Transform 8.0 "/7
  data_in_tlast/1 -> [FFT_IN_tlast], "Fast Fourier Transform 8.0 "/8
  Convert/1 -> Gateway Out9/1, "Fast Fourier Transform 8.0 "/3
  Gateway Out7/1 -> FFT Ctrl/3  "IN tlast"
  Gateway Out6/1 -> FFT Status/5  "tlast_missing"
  Gateway Out5/1 -> FFT Status/4  "tlast_unexpected"
  Gateway Out4/1 -> FFT Status/3  "frame started"
  Gateway Out1/1 -> FFT Ctrl/1  "IN tready"
  Gateway Out/1 -> FFT Ctrl/2  "IN tvalid"
  [FFT_IN_data_tready] -> data_in_tready/1
  [FFT_OUT_xk_re] -> I out/1
  [FFT_OUT_xk_im] -> Q out/1
  [FFT_OUT_data_tvalid] -> data_out_tvalid/1
  [FFT_OUT_data_tlast] -> data_out_tlast/1
  Gateway Out3/1 -> FFT Ctrl/4  "OUT tvalid"
  Gateway Out10/1 -> FFT Ctrl/5  "OUT tlast"
  Gateway Out11/1 -> FFT Ctrl/6  "OUT xkindex"
  Gateway Out12/1 -> FFT Status/2  "IN tlast"
  Gateway Out13/1 -> FFT Status/1  "IN tvalid"
  [FFT_IN_data_tready] -> Gateway Out1/1
  [FFT_IN_tvalid] -> Gateway Out/1
  [FFT_IN_tlast] -> Gateway Out7/1
  [FFT_OUT_data_tvalid] -> Gateway Out3/1
  [FFT_OUT_data_tlast] -> Gateway Out10/1
  [FFT_OUT_xk_index] -> Gateway Out11/1
  [FFT_IN_tvalid] -> Gateway Out13/1
  [FFT_IN_tlast] -> Gateway Out12/1
  [FFT_event_frame_started] -> Gateway Out4/1
  [FFT_event_tlast_unexpected] -> Gateway Out5/1
  [FFT_event_tlast_missnig] -> Gateway Out6/1
  [FFT_OUT_xk_index] -> data_xk_index/1, Reinterpret/1
  Constant/1 -> FFT Ctrl/7
  Constant5/1 -> FFT Ctrl/8
  Gateway Out15/1 -> FFT Status/8  "OUT tvalid"
  [FFT_OUT_data_tvalid] -> Gateway Out15/1
  Constant1/1 -> "Fast Fourier Transform 8.0 "/2
  Constant4/1 -> "Fast Fourier Transform 8.0 "/4
  Q in/1 -> "Fast Fourier Transform 8.0 "/5
  I in/1 -> "Fast Fourier Transform 8.0 "/6
  Constant2/1 -> "Fast Fourier Transform 8.0 "/9
  Inverter/1 -> "Fast Fourier Transform 8.0 "/11
  Constant3/1 -> "Fast Fourier Transform 8.0 "/10
  "Fast Fourier Transform 8.0 "/1 -> [FFT_config_tready]
  "Fast Fourier Transform 8.0 "/2 -> [FFT_IN_data_tready]
  "Fast Fourier Transform 8.0 "/3 -> [FFT_status_tvalid]
  "Fast Fourier Transform 8.0 "/4 -> [FFT_status_tdata_ovflo]
  "Fast Fourier Transform 8.0 "/5 -> [FFT_OUT_xk_im]
  "Fast Fourier Transform 8.0 "/6 -> [FFT_OUT_xk_re]
  "Fast Fourier Transform 8.0 "/7 -> [FFT_data_tuser_ovflo]
  "Fast Fourier Transform 8.0 "/8 -> [FFT_OUT_xk_index]
  "Fast Fourier Transform 8.0 "/9 -> [FFT_OUT_data_tvalid]
  "Fast Fourier Transform 8.0 "/10 -> [FFT_OUT_data_tlast]
  "Fast Fourier Transform 8.0 "/11 -> [FFT_event_frame_started]
  "Fast Fourier Transform 8.0 "/12 -> [FFT_event_tlast_unexpected]
  "Fast Fourier Transform 8.0 "/13 -> [FFT_event_tlast_missnig]
  [FFT_data_tuser_ovflo] -> Gateway Out2/1
  Gateway Out2/1 -> FFT Status/6  "tuser_ovflo"
  Gateway Out14/1 -> FFT Status/7  "tdata_ovflo"
  [FFT_status_tdata_ovflo] -> Gateway Out14/1
  "Fast Fourier Transform 8.0 "/14 -> [FFT_event_fft_overflow]
  Reinterpret/1 -> Convert1/1

== system wlan_phy_tx_pmd/FFT/S-R Latch2 ==
  S : Inport
  R : Inport  Port=2
  Constant1 : xbsIndex_r4/Constant  const=1  gui_display_data_type=Fixed-point  arith_type=Boolean  n_bits=1  bin_pt=0  preci_type=Single  exp_width=8  frac_width=24  explicit_period=off  period=1  equ=P=C  opselect=C  inp2=PCIN>>17  opr=+  inp1=P  carry=CIN  dbl_ovrd=off  block_type=constant
      settings: block_version=VER_STRING_GOES_HERE
  Convert1 : xbsIndex_r4/Convert  gui_display_data_type=Boolean  arith_type=Boolean  n_bits=1  bin_pt=0  float_type=Single  exp_bits=8  fraction_bits=24  quantization=Truncate  overflow=Wrap  en=off  latency=0  dbl_ovrd=off  pipeline=off  block_type=convert
  Convert2 : xbsIndex_r4/Convert  gui_display_data_type=Boolean  arith_type=Boolean  n_bits=1  bin_pt=0  float_type=Single  exp_bits=8  fraction_bits=24  quantization=Truncate  overflow=Wrap  en=off  latency=0  dbl_ovrd=off  pipeline=off  block_type=convert
  Register2 : xbsIndex_r4/Register  init=0  rst=on  en=on  dbl_ovrd=off  block_type=register
      settings: xl_area=[1 1 0 0 0 0 0]  block_version=VER_STRING_GOES_HERE
  Q : Outport
  wires:
  Convert2/1 -> Register2/3
  Convert1/1 -> Register2/2
  Constant1/1 -> Register2/1
  R/1 -> Convert1/1
  Register2/1 -> Q/1
  S/1 -> Convert2/1

== system wlan_phy_tx_pmd/FFT/valid only ==
  ready : Inport
  valid : Inport  Port=2
  D : Inport  Port=3
  Constant4 : xbsIndex_r4/Constant  const=-1  gui_display_data_type=Fixed-point  arith_type=Signed (2's comp)  n_bits=2  bin_pt=0  preci_type=Single  exp_width=8  frac_width=24  explicit_period=on  period=1  equ=P=C  opselect=C  inp2=PCIN>>17  opr=+  inp1=P  carry=CIN  dbl_ovrd=off  block_type=constant
  Logical : xbsIndex_r4/Logical  logical_function=AND  inputs=2  en=off  latency=0  precision=Full  arith_type=Unsigned  n_bits=16  bin_pt=0  align_bp=on  dbl_ovrd=off  block_type=logical
  Mux : xbsIndex_r4/Mux  inputs=2  en=off  latency=0  precision=Full  arith_type=Unsigned  n_bits=16  bin_pt=14  quantization=Truncate  overflow=Wrap  dbl_ovrd=off  block_type=mux
  Q : Outport
  wires:
  Mux/1 -> Q/1
  D/1 -> Mux/3
  valid/1 -> Logical/2
  ready/1 -> Logical/1
  Constant4/1 -> Mux/2
  Logical/1 -> Mux/1

== system wlan_phy_tx_pmd/FFT/valid only1 ==
  D : Inport
  valid : Inport  Port=2
  Constant4 : xbsIndex_r4/Constant  const=-1  gui_display_data_type=Fixed-point  arith_type=Signed (2's comp)  n_bits=2  bin_pt=0  preci_type=Single  exp_width=8  frac_width=24  explicit_period=on  period=1  equ=P=C  opselect=C  inp2=PCIN>>17  opr=+  inp1=P  carry=CIN  dbl_ovrd=off  block_type=constant
  Mux : xbsIndex_r4/Mux  inputs=2  en=off  latency=0  precision=Full  arith_type=Unsigned  n_bits=16  bin_pt=14  quantization=Truncate  overflow=Wrap  dbl_ovrd=off  block_type=mux
  Q : Outport
  wires:
  Constant4/1 -> Mux/2
  valid/1 -> Mux/1
  D/1 -> Mux/3
  Mux/1 -> Q/1

== system wlan_phy_tx_pmd/FIFO/I/Q Concat ==
  I : Inport
  Q : Inport  Port=2
  Concat : xbsIndex_r4/Concat  num_inputs=2  dbl_ovrd=off  block_type=concat
  Reinterpret : xbsIndex_r4/Reinterpret  force_arith_type=on  arith_type=Unsigned  force_bin_pt=on  bin_pt=0  block_type=reinterpret
  Reinterpret1 : xbsIndex_r4/Reinterpret  force_arith_type=on  arith_type=Unsigned  force_bin_pt=on  bin_pt=0  block_type=reinterpret
  IQ : Outport
  wires:
  Reinterpret/1 -> Concat/1
  Reinterpret1/1 -> Concat/2
  I/1 -> Reinterpret/1
  Concat/1 -> IQ/1
  Q/1 -> Reinterpret1/1

== system wlan_phy_tx_pmd/FIFO/I/Q Slice ==
  IQ : Inport
  Reinterpret2 : xbsIndex_r4/Reinterpret  force_arith_type=on  arith_type="Signed  (2's comp)"  force_bin_pt=on  bin_pt=15  block_type=reinterpret
  Reinterpret3 : xbsIndex_r4/Reinterpret  force_arith_type=on  arith_type="Signed  (2's comp)"  force_bin_pt=on  bin_pt=15  block_type=reinterpret
  Slice : xbsIndex_r4/Slice  nbits=16  boolean_output=off  mode=Upper Bit Location + Width  bit1=0  base1=MSB of Input  bit0=0  base0=LSB of Input  dbl_ovrd=off  block_type=slice
  Slice1 : xbsIndex_r4/Slice  nbits=16  boolean_output=off  mode=Lower Bit Location + Width  bit1=0  base1=MSB of Input  bit0=0  base0=LSB of Input  dbl_ovrd=off  block_type=slice
  I : Outport
  Q : Outport  Port=2
  wires:
  Reinterpret3/1 -> Q/1
  Reinterpret2/1 -> I/1
  IQ/1 -> Slice/1, Slice1/1
  Slice1/1 -> Reinterpret3/1
  Slice/1 -> Reinterpret2/1
